simulink model "Interface_Model"  (R2019b)
settings: Solver=FixedStepDiscrete  StartTime=0.0  StopTime=inf  RelTol=1e-3  EnableMultiTasking=on
InitFcn:
  | modelSettings
undefined symbols (not defined in the file): Fs, ip
libraries: ad936xlib x2, gm_combinedTxRx_ExternalMode_lib x1
settings Model: SimulationMode=external  Creator=tcollins  LastModifiedBy=bhisma
settings SolverCC: PositivePriorityOrder=on
settings DataIOCC: ReturnWorkspaceOutputs=off
settings OptimizationCC: BlockReduction=off  ConditionallyExecuteInputs=off  PassReuseOutputArgsAs=Individual arguments  MaxStackSize=64  EfficientTunableParamExpr=on
settings DebuggingCC: AlgebraicLoopMsg=error  SingleTaskRateTransMsg=error  ParameterTunabilityLossMsg=error  ArithmeticOperatorsInVariantConditions=warning
settings HardwareCC: ProdBitPerPointer=32  ProdBitPerSizeT=32  ProdBitPerPtrDiffT=32  ProdLargestAtomicInteger=Long  ProdLargestAtomicFloat=Double  ProdWordSize=32  ProdLongLongMode=on  ProdHWDeviceType=ARM Compatible->ARM Cortex  TargetLargestAtomicInteger=Long  TargetLargestAtomicFloat=Double  TargetIntDivRoundTo=Zero  TargetEndianess=LittleEndian  TargetHWDeviceType=ARM Compatible->ARM Cortex
settings SFSimCC: SimUseLocalCustomCode=off  MATLABDynamicMemAlloc=off  CustomCodeUndefinedFunction=UseInterfaceOnly
settings RTWCC: SystemTargetFile=ert.tlc  HardwareBoard=Xilinx Zynq-7000 Based IIO Radio  TLCOptions="-aInlineSetEventsForThisBaseRateFcn=TLC_FALSE -aSuppressMultiTaskScheduler=TLC_FALSE  -aRateBasedStepFcn=0"  TemplateMakefile=ert_default_tmf  RTWUseLocalCustomCode=off  Toolchain=Xilinx Software Development Kit (SDK)  IncludeHyperlinkInReport=on
settings CodeAppCC: ForceParamTrailComments=on  IgnoreCustomStorageClasses=off  OperatorAnnotations=on  SimulinkDataObjDesc=on  SFDataObjDesc=on  InsertBlockDesc=on

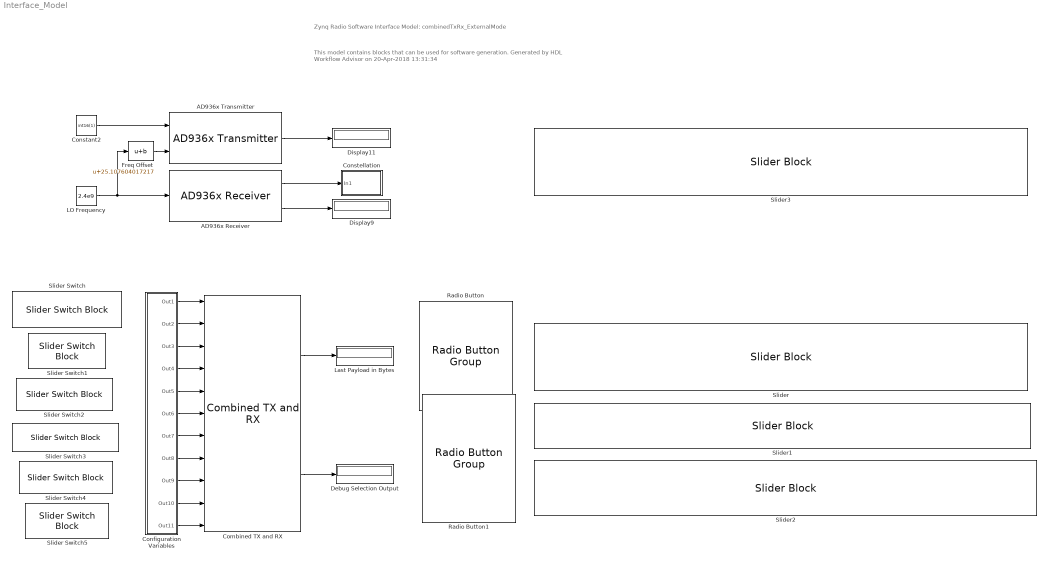
== system Interface_Model ==
  note: Zynq Radio Software Interface Model: combinedTxRx_ExternalMode
  note: This model contains blocks that can be used for software generation.
      |
      | Generated by HDL Workflow Advisor on 20-Apr-2018 13:31:34
  AD936x Receiver : ad936xlib/AD936x Receiver  SourceLibraryInfo="This block requires <a href=\"http://www.mathworks.com/hardware-support/rtl-sdr.html\">Communications System Toolbox Support Package for RTL-SDR Radio</a>"  IPAddress=192.168.3.2  uri=ip:10.0.0.200  CenterFrequencySource=Input Port  CenterFrequency=2.4e9  GainSource=AGC Slow Attack  GainSourceBlock=AGC Slow Attack  Gain=10  ChannelMapping=1  BasebandSampleRate=1e6  OutputDataType=int16  SamplesPerFrame=20000  OverflowOutputPort=on  EnableBurstMode=off  NumFramesInBurst=1  ShowAdvancedProperties=off  UseCustomFilter=off  filtPathRates=[ 737280000, 11520000, 3840000, 1920000, 960000, 240000 ]  filtCoefficients=round( fir1( 127, 0.75 )*2^15*10^1.2 )  filtCoefficientSize=128  filtDecimInterpFactor=4  filtGain=-12  filtRFBandwidth=18e6  filterConfigStruct=struct()  EnableQuadratureCorrection=on  EnableRFDCCorrection=on  EnableBasebandDCCorrection=on  OverrideSampleTime=off  SampleTime=0.02  DataTimeout=Inf  ENSMPinControlMode=None  BISTLoopbackMode=Disabled  BISTToneInject=Disabled  BISTSignalGen=PRBS  BISTToneFreq=Fs/32  BISTToneLevel=0
      settings: SourceProductName=Communications Toolbox Support Package for Xilinx Zynq-Based Radio
  AD936x Transmitter : ad936xlib/AD936x Transmitter  SourceLibraryInfo="This block requires <a href=\"http://www.mathworks.com/hardware-support/rtl-sdr.html\">Communications System Toolbox Support Package for RTL-SDR Radio</a>"  IPAddress=192.168.3.2  uri=ip:10.0.0.200  CenterFrequencySource=Input Port  CenterFrequency=2.4e9  GainSource=Dialog  Gain=-10  ChannelMapping=1  BasebandSampleRate=1e6  UnderflowOutputPort=on  ShowAdvancedProperties=off  UseCustomFilter=off  filtPathRates=[ 737280000, 11520000, 3840000, 1920000, 960000, 240000 ]  filtCoefficients=round( fir1( 127, 0.75 )*2^15*10^1.2 )  filtCoefficientSize=128  filtDecimInterpFactor=4  filtGain=-12  filtRFBandwidth=18e6  filterConfigStruct=struct()  DataSourceSelect=Input Port  DDSTone1Freq=5e3  DDSTone2Freq=10e3  DDSTone1Scale=0.5  DDSTone2Scale=0.25  DataTimeout=Inf  ENSMPinControlMode=None  BISTLoopbackMode=Disabled  BISTToneInject=Disabled  BISTSignalGen=PRBS  BISTToneFreq=Fs/32  BISTToneLevel=0
      settings: SourceProductName=Communications Toolbox Support Package for Xilinx Zynq-Based Radio
  Combined TX and RX : gm_combinedTxRx_ExternalMode_lib/Combined TX and RX
  Configuration Variables : Subsystem
  Constant2 : Constant  Value=int16(1)  SampleTime=1/500
  Constellation : Subsystem
  Debug Selection Output : Display
  Display11 : Display
  Display9 : Display
  Freq Offset : Bias  Bias=25.107604017217
  LO Frequency : Constant  Value=2.4e9  SampleTime=1/500
  Last Payload in Bytes : Display
  Radio Button : RadioButtonGroup  SelectedLabel=After Frequency Recovery  ButtonGroupName=Constellation Data Source
      settings: Values={{'After SRRC', 'After Timing Recovery', 'After Frequency Recovery', 'After EQ'}, [1 2 3 4]}
  Radio Button1 : RadioButtonGroup  SelectedLabel=CRC Errors  ButtonGroupName=Constellation Data Source
      settings: Values={{'Timing Lock', 'Peaks Found', 'Freq Lock', 'Header Failures', 'CRC Errors', 'Packet Count', 'Last Payload Length'}, [0 1 2 3 4 5 6]}
  Slider : SliderBlock  ScaleMin=1  TickInterval=9
  Slider Switch{,1..5} (6 alike) : SliderSwitchBlock
  Slider1 : SliderBlock  ScaleMin=20  ScaleMax=500  TickInterval=40
  Slider2 : SliderBlock  ScaleMax=40
  Slider3 : SliderBlock  ScaleMin=-1000  ScaleMax=1000  TickInterval=100
  wires:
  Configuration Variables/2(Out2) -> Combined TX and RX/2
  Combined TX and RX/2 -> Debug Selection Output/1
  Configuration Variables/8(Out8) -> Combined TX and RX/8
  Configuration Variables/7(Out7) -> Combined TX and RX/7
  Configuration Variables/1(Out1) -> Combined TX and RX/1
  Configuration Variables/5(Out5) -> Combined TX and RX/5
  Configuration Variables/10(Out10) -> Combined TX and RX/10
  Configuration Variables/3(Out3) -> Combined TX and RX/3
  Configuration Variables/9(Out9) -> Combined TX and RX/9
  Configuration Variables/6(Out6) -> Combined TX and RX/6
  Combined TX and RX/1 -> Last Payload in Bytes/1
  Configuration Variables/4(Out4) -> Combined TX and RX/4
  Configuration Variables/11(Out11) -> Combined TX and RX/11
  AD936x Transmitter/1 -> Display11/1
  AD936x Receiver/2 -> Display9/1
  Constant2/1 -> AD936x Transmitter/1
  AD936x Receiver/1 -> Constellation/1(In1)
  LO Frequency/1 -> Freq Offset/1, AD936x Receiver/1
  Freq Offset/1 -> AD936x Transmitter/2

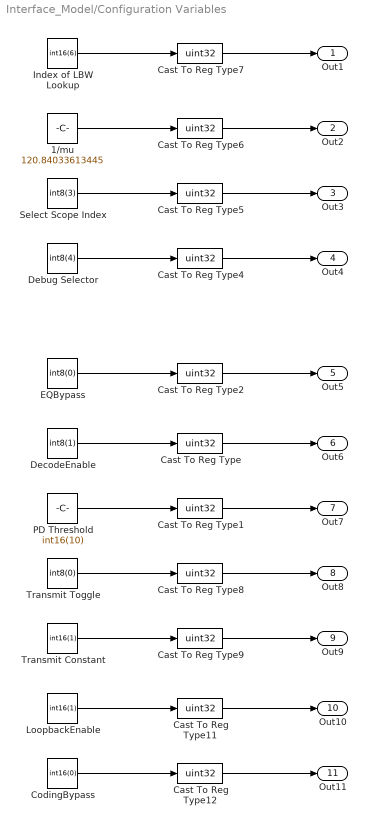
== system Interface_Model/Configuration Variables ==
  1/mu : Constant  Value=120.84033613445  OutDataTypeStr=int16  SampleTime=1/500
  Cast To Reg Type{,1..2,4..9,11..12} (11 alike) : DataTypeConversion  OutDataTypeStr=uint32
  CodingBypass : Constant  Value=int16(0)  SampleTime=1/500
  Debug Selector : Constant  Value=int8(4)  SampleTime=1/500
  DecodeEnable : Constant  Value=int8(1)  SampleTime=1/500
  EQBypass : Constant  Value=int8(0)  SampleTime=1/500
  Index of LBW Lookup : Constant  Value=int16(6)  SampleTime=1/500
  LoopbackEnable : Constant  Value=int16(1)  SampleTime=1/500
  PD Threshold : Constant  Value=int16(10)  SampleTime=1/500
  Select Scope Index : Constant  Value=int8(3)  SampleTime=1/500
  Transmit Constant : Constant  Value=int16(1)  SampleTime=1/500
  Transmit Toggle : Constant  Value=int8(0)  SampleTime=1/500
  Out1 : Outport  VectorParamsAs1DForOutWhenUnconnected=off
  Out2 : Outport  Port=2  VectorParamsAs1DForOutWhenUnconnected=off
  Out3 : Outport  Port=3  VectorParamsAs1DForOutWhenUnconnected=off
  Out4 : Outport  Port=4  VectorParamsAs1DForOutWhenUnconnected=off
  Out5 : Outport  Port=5  VectorParamsAs1DForOutWhenUnconnected=off
  Out6 : Outport  Port=6  VectorParamsAs1DForOutWhenUnconnected=off
  Out7 : Outport  Port=7  VectorParamsAs1DForOutWhenUnconnected=off
  Out8 : Outport  Port=8  VectorParamsAs1DForOutWhenUnconnected=off
  Out9 : Outport  Port=9  VectorParamsAs1DForOutWhenUnconnected=off
  Out10 : Outport  Port=10  VectorParamsAs1DForOutWhenUnconnected=off
  Out11 : Outport  Port=11  VectorParamsAs1DForOutWhenUnconnected=off
  wires:
  1/mu/1 -> Cast To Reg Type6/1
  Index of LBW Lookup/1 -> Cast To Reg Type7/1
  Select Scope Index/1 -> Cast To Reg Type5/1
  Debug Selector/1 -> Cast To Reg Type4/1
  EQBypass/1 -> Cast To Reg Type2/1
  DecodeEnable/1 -> Cast To Reg Type/1
  PD Threshold/1 -> Cast To Reg Type1/1
  Cast To Reg Type1/1 -> Out7/1
  Cast To Reg Type/1 -> Out6/1
  Cast To Reg Type2/1 -> Out5/1
  Cast To Reg Type4/1 -> Out4/1
  Cast To Reg Type5/1 -> Out3/1
  Cast To Reg Type6/1 -> Out2/1
  Cast To Reg Type7/1 -> Out1/1
  Transmit Toggle/1 -> Cast To Reg Type8/1
  Transmit Constant/1 -> Cast To Reg Type9/1
  Cast To Reg Type9/1 -> Out9/1
  Cast To Reg Type8/1 -> Out8/1
  LoopbackEnable/1 -> Cast To Reg Type11/1
  Cast To Reg Type11/1 -> Out10/1
  CodingBypass/1 -> Cast To Reg Type12/1
  Cast To Reg Type12/1 -> Out11/1

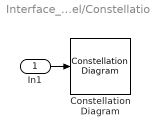
== system Interface_Model/Constellation ==
  In1 : Inport
  Constellation Diagram : ConstellationDiagram
  wires:
  In1/1 -> Constellation Diagram/1
